simulink model "model"  (R2022b)
settings: Solver=VariableStepAuto  StartTime=0.0  StopTime=15  RelTol=1e-3
libraries: neural x114, simulink x4
(part 3 of 4)

== system model/level=2，训练时间15s，隐藏层30/Layer 2/LW{2,1} ==
  "ad{2,1}" : Inport  PortDimensions=30
      mask Display: e = 0.06;c1 = [120 230 180]/255;c2 = ([120 230 180]+0)/(256+128);c3 = ([120 230 180]+128)/(256+128);patch([0 1 1 0],[0 0 1 1],c1);patch([0 1 1 1-e 1-e 0+e],[0 0 1 1-e 0+e 0+e],c2);patch([0 0 1 1-e 0+e 0+e],[0 1 1 1-e 1-e 0+e],c3);plot([0 1 1 0 0],[0 0 1 1 0]);
  "IW{2,1}(1,:)'" : Constant  Value=[-0.00017015661933175867700888950206916661045397631824016571044921875;-4.93025601643951106906223202930306115376879461109638214111328125e-05;-0.0007115142662295552249129837463215153547935187816619873046875;0.450465904697785302079893199334037490189075469970703125;-0.00035970417057819303353893847230438041151501238346099853515625;-0.00046544183662747154288374940023231829400174319744110107421875;-0.000876727493122407487875780152108973197755403816699981689453125;0.0002626128599686000327818879984675959349260665476322174072265625;0.3370860472746011193834192454232834279537200927734375;-0.00158890258031656596109104651048937739687971770763397216796875;-0.860928350444378320815985716762952506542205810546875;-2.2868367123550593163379407446456070829299278557300567626953125e-05;3.394770767892958175139528353980722386040724813938140869140625e-05;3.60748119126446740024920234457539436334627680480480194091796875e-05;0.00010252607091006281565294389057640955797978676855564117431640625;0.0003053396075934432349514857651939792049233801662921905517578125;-0.0208847293595013257239134674136948888190090656280517578125;0.00018090783389240641491901850912427107687108218669891357421875;0.0035955382769562497201343287400732151581905782222747802734375;2.9147343262242141341718248970238391848397441208362579345703125e-05;-1.044255751802114051685066442587412893772125244140625;7.6663907290150487723601191447642122511751949787139892578125e-05;1.1612112621581929250424991550971753895282745361328125;8.69004399139240257636529474183362253825180232524871826171875e-05;-0.00089584410815050333383446901081015312229283154010772705078125;0.000972428946461849873228455720663987449370324611663818359375;-0.55852210608613506170883056256570853292942047119140625;0.00014495112667725106102116494621867559544625692069530487060546875;-0.0011652466891173842399032078986920168972574174404144287109375;-0.00063093431305860973000443348013277500285767018795013427734375]
      mask Display: e = 0.06;c1 = [120 150 230]/255;c2 = ([120 150 230]+0)/383;c3 = ([120 150 230]+128)/383;patch([0 1 1 0],[0 0 1 1],c1);patch([0 1 1 1-e 1-e 0+e],[0 0 1 1-e 0+e 0+e],c2);patch([0 0 1 1-e 0+e 0+e],[0 1 1 1-e 1-e 0+e],c3);plot([0 1 1 0 0],[0 0 1 1 0]);disp('weights');
  "IW{2,1}(2,:)'" : Constant  Value=[5.38258205100171352648109890370875518783577717840671539306640625e-05;-0.00013672751288354225720177159697499291723943315446376800537109375;0.000678841755202407026725808236733428202569484710693359375;-0.98479814361060780125711744403815828263759613037109375;0.0002569134171630268310103362150442762867896817624568939208984375;0.000626265400513533886280026496962136661750264465808868408203125;0.00056349774478808563153708899307048341142944991588592529296875;-0.000564491732790600199420882887579864473082125186920166015625;-1.2396930325476953616004038849496282637119293212890625;0.00152451867466346234654406277542193492990918457508087158203125;-0.202489611993786733368239083574735559523105621337890625;-0.0004488496149839809744482022058065240344149060547351837158203125;0.0001848497058731152806014541578605303584481589496135711669921875;0.00013099649124499862236185865338455869277822785079479217529296875;-0.000290407580426385570314395945246133123873732984066009521484375;-0.0002539432359679540704248956739519371694768778979778289794921875;0.0241381257840159908767407870300303329713642597198486328125;-0.00025981285471116284668813278813104261644184589385986328125;-0.004254317985620206625518857634915548260323703289031982421875;7.9434875059497178835000996688364693909534253180027008056640625e-05;0.8138138000844878927608760932344011962413787841796875;-0.0002077032004498433558591086178779505644342862069606781005859375;-0.0224187640494880081887263401085874647833406925201416015625;9.7974639247613346903879871785392197125474922358989715576171875e-05;0.00107277211369045423483559176247581490315496921539306640625;-0.00023836869626189699272918176564672876338590867817401885986328125;0.15422244230446391366484704121830873191356658935546875;-0.000510323222761460237699437936242929936270229518413543701171875;0.0013619494124274072154034964654556461027823388576507568359375;0.00018567701461944481947617668904371157623245380818843841552734375]
      mask Display: e = 0.06;c1 = [120 150 230]/255;c2 = ([120 150 230]+0)/383;c3 = ([120 150 230]+128)/383;patch([0 1 1 0],[0 0 1 1],c1);patch([0 1 1 1-e 1-e 0+e],[0 0 1 1-e 0+e 0+e],c2);patch([0 0 1 1-e 0+e 0+e],[0 1 1 1-e 1-e 0+e],c3);plot([0 1 1 0 0],[0 0 1 1 0]);disp('weights');
  Mux : Mux  Inputs=2
      mask Display: e = 0.06;c1 = [120 150 230]/255;c2 = ([120 150 230]+0)/383;c3 = ([120 150 230]+128)/383;patch([0 1 1 0],[0 0 1 1],c1);patch([0 1 1 1-e 1-e 0+e],[0 0 1 1-e 0+e 0+e],c2);patch([0 0 1 1-e 0+e 0+e],[0 1 1 1-e 1-e 0+e],c3);plot([0 1 1 0 0],[0 0 1 1 0]);disp('Mux');
  dotprod1 : neural/Weight Functions/dotprod
  dotprod2 : neural/Weight Functions/dotprod
  "lz{2,1}" : Outport
      mask Display: e = 0.06;c1 = [120 230 180]/255;c2 = ([120 230 180]+0)/(256+128);c3 = ([120 230 180]+128)/(256+128);patch([0 1 1 0],[0 0 1 1],c1);patch([0 1 1 1-e 1-e 0+e],[0 0 1 1-e 0+e 0+e],c2);patch([0 0 1 1-e 0+e 0+e],[0 1 1 1-e 1-e 0+e],c3);plot([0 1 1 0 0],[0 0 1 1 0]);
  wires:
  "IW{2,1}(1,:)'"/1 -> dotprod1/1
  "ad{2,1}"/1 -> dotprod1/2, dotprod2/2
  dotprod1/1 -> Mux/1
  "IW{2,1}(2,:)'"/1 -> dotprod2/1
  dotprod2/1 -> Mux/2
  Mux/1 -> "lz{2,1}"/1

== system model/level=3，训练时间15s，隐藏层15/Layer 1/Delays 1 ==
  "p{1}" : Inport  PortDimensions=12
      mask Display: e = 0.06;c1 = [120 230 180]/255;c2 = ([120 230 180]+0)/(256+128);c3 = ([120 230 180]+128)/(256+128);patch([0 1 1 0],[0 0 1 1],c1);patch([0 1 1 1-e 1-e 0+e],[0 0 1 1-e 0+e 0+e],c2);patch([0 0 1 1-e 0+e 0+e],[0 1 1 1-e 1-e 0+e],c3);plot([0 1 1 0 0],[0 0 1 1 0]);
  mux : Mux  Inputs=1
      mask Display: e = 0.06;c1 = [120 150 230]/255;c2 = ([120 150 230]+0)/383;c3 = ([120 150 230]+128)/383;patch([0 1 1 0],[0 0 1 1],c1);patch([0 1 1 1-e 1-e 0+e],[0 0 1 1-e 0+e 0+e],c2);patch([0 0 1 1-e 0+e 0+e],[0 1 1 1-e 1-e 0+e],c3);plot([0 1 1 0 0],[0 0 1 1 0]);disp('Mux')
  "pd{1,1}" : Outport
      mask Display: e = 0.06;c1 = [120 230 180]/255;c2 = ([120 230 180]+0)/(256+128);c3 = ([120 230 180]+128)/(256+128);patch([0 1 1 0],[0 0 1 1],c1);patch([0 1 1 1-e 1-e 0+e],[0 0 1 1-e 0+e 0+e],c2);patch([0 0 1 1-e 0+e 0+e],[0 1 1 1-e 1-e 0+e],c3);plot([0 1 1 0 0],[0 0 1 1 0]);
  wires:
  "p{1}"/1 -> mux/1
  mux/1 -> "pd{1,1}"/1

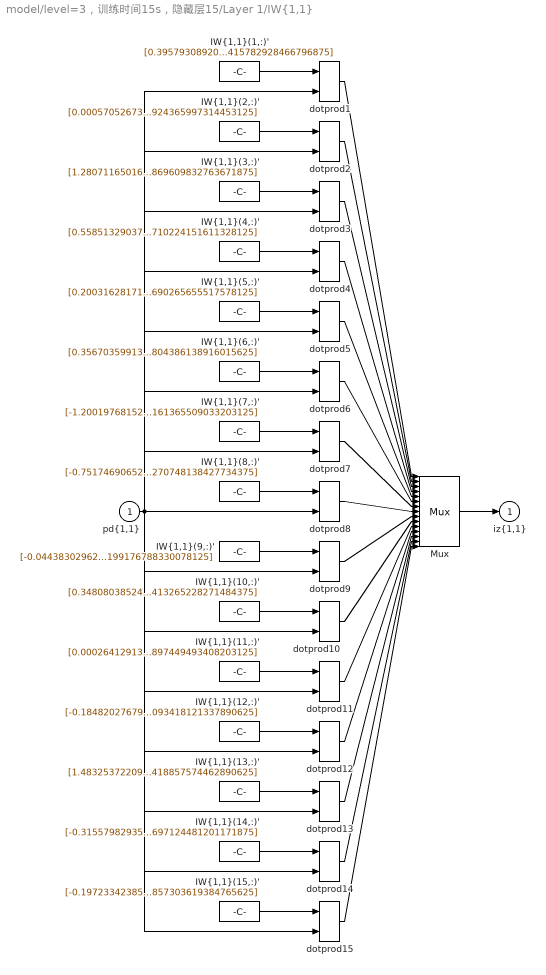
== system model/level=3，训练时间15s，隐藏层15/Layer 1/IW{1,1} ==
  "pd{1,1}" : Inport  PortDimensions=12
      mask Display: e = 0.06;c1 = [120 230 180]/255;c2 = ([120 230 180]+0)/(256+128);c3 = ([120 230 180]+128)/(256+128);patch([0 1 1 0],[0 0 1 1],c1);patch([0 1 1 1-e 1-e 0+e],[0 0 1 1-e 0+e 0+e],c2);patch([0 0 1 1-e 0+e 0+e],[0 1 1 1-e 1-e 0+e],c3);plot([0 1 1 0 0],[0 0 1 1 0]);
  "IW{1,1}(1,:)'" : Constant  Value=[0.3957930892014740464901478844694793224334716796875;0.086698682741434496268340126334805972874164581298828125;0.057978420610327340012357666410025558434426784515380859375;-0.11708503503631663422712705369121977128088474273681640625;0.5757139566791853457772276669857092201709747314453125;0.100001463605383589250408249426982365548610687255859375;-0.360494014120566863557115766525384970009326934814453125;0.331018839262216479912837030497030355036258697509765625;0.67861213442945389484606266705668531358242034912109375;1.62287556740570426683234472875483334064483642578125;1.1914706007323612180215377520653419196605682373046875;1.5007337994294249750026892797905020415782928466796875]
      mask Display: e = 0.06;c1 = [120 150 230]/255;c2 = ([120 150 230]+0)/383;c3 = ([120 150 230]+128)/383;patch([0 1 1 0],[0 0 1 1],c1);patch([0 1 1 1-e 1-e 0+e],[0 0 1 1-e 0+e 0+e],c2);patch([0 0 1 1-e 0+e 0+e],[0 1 1 1-e 1-e 0+e],c3);plot([0 1 1 0 0],[0 0 1 1 0]);disp('Weights');
  "IW{1,1}(10,:)'" : Constant  Value=[0.348080385247078794019870429110596887767314910888671875;-2.255687632373656992257338060881011188030242919921875;-0.8917795900077691850782457549939863383769989013671875;1.1584959880156178169130498645245097577571868896484375;-0.81101211177083321057779130569542758166790008544921875;0.062260937313953899907570388450039899908006191253662109375;0.53574182001364734073689533033757470548152923583984375;-0.2128709739492778696412500494261621497571468353271484375;-0.46279511588180832770689221433713100850582122802734375;-0.34533064631210741435296540657873265445232391357421875;-1.10111951608478175756999917211942374706268310546875;1.12329307949009571387932737707160413265228271484375]
      mask Display: e = 0.06;c1 = [120 150 230]/255;c2 = ([120 150 230]+0)/383;c3 = ([120 150 230]+128)/383;patch([0 1 1 0],[0 0 1 1],c1);patch([0 1 1 1-e 1-e 0+e],[0 0 1 1-e 0+e 0+e],c2);patch([0 0 1 1-e 0+e 0+e],[0 1 1 1-e 1-e 0+e],c3);plot([0 1 1 0 0],[0 0 1 1 0]);disp('Weights');
  "IW{1,1}(11,:)'" : Constant  Value=[0.0002641291373141290798991220878377816916326992213726043701171875;1.69280234455796972669640310105165781351388432085514068603515625e-05;0.00059389072570711367270168690168929970241151750087738037109375;0.000817075702284870562970564566995790301007218658924102783203125;-0.0002773395932363266892621556092279888616758398711681365966796875;0.000419950685599850752176276369453944425913505256175994873046875;1.7279375298931984872297107358463108539581298828125;1.1830523399036094733816071311593987047672271728515625;0.385067347353057087833150262667913921177387237548828125;0.47274192642379031514821008386206813156604766845703125;-0.85106281929793781149129472396452911198139190673828125;-0.75527215984610063248538835978251881897449493408203125]
      mask Display: e = 0.06;c1 = [120 150 230]/255;c2 = ([120 150 230]+0)/383;c3 = ([120 150 230]+128)/383;patch([0 1 1 0],[0 0 1 1],c1);patch([0 1 1 1-e 1-e 0+e],[0 0 1 1-e 0+e 0+e],c2);patch([0 0 1 1-e 0+e 0+e],[0 1 1 1-e 1-e 0+e],c3);plot([0 1 1 0 0],[0 0 1 1 0]);disp('Weights');
  "IW{1,1}(12,:)'" : Constant  Value=[-0.1848202767977935312426751579550909809768199920654296875;0.012338003346249258596056819214936695061624050140380859375;0.09999923402391842908176755599924945272505283355712890625;-0.29923701483788744948100202236673794686794281005859375;-0.2017986819280386534547488963653449900448322296142578125;-0.00197252352955649447319164124792223447002470493316650390625;-1.370526397980648791730118318810127675533294677734375;-0.58819022085026995139145356006338261067867279052734375;-0.8059703463854150928824537913897074759006500244140625;0.602810685508602173143799518584273755550384521484375;0.87530414850278026595020719469175674021244049072265625;-0.00901182558217848185544429640003727399744093418121337890625]
      mask Display: e = 0.06;c1 = [120 150 230]/255;c2 = ([120 150 230]+0)/383;c3 = ([120 150 230]+128)/383;patch([0 1 1 0],[0 0 1 1],c1);patch([0 1 1 1-e 1-e 0+e],[0 0 1 1-e 0+e 0+e],c2);patch([0 0 1 1-e 0+e 0+e],[0 1 1 1-e 1-e 0+e],c3);plot([0 1 1 0 0],[0 0 1 1 0]);disp('Weights');
  "IW{1,1}(13,:)'" : Constant  Value=[1.4832537220993196047658102543209679424762725830078125;0.206296960918707750209932783036492764949798583984375;-0.86180429757193277584548241065931506454944610595703125;-0.52558132261974599419573905834113247692584991455078125;1.22454643654238193306582616060040891170501708984375;0.64085174940409228572235633691889233887195587158203125;1.730080809760341953307261064765043556690216064453125;4.73501628594810686223581797094084322452545166015625;2.770509814033699225177542757592163980007171630859375;2.547005844747089131629991243244148790836334228515625;2.063288887946004734885718789882957935333251953125;0.56434669201611209476965314024710096418857574462890625]
      mask Display: e = 0.06;c1 = [120 150 230]/255;c2 = ([120 150 230]+0)/383;c3 = ([120 150 230]+128)/383;patch([0 1 1 0],[0 0 1 1],c1);patch([0 1 1 1-e 1-e 0+e],[0 0 1 1-e 0+e 0+e],c2);patch([0 0 1 1-e 0+e 0+e],[0 1 1 1-e 1-e 0+e],c3);plot([0 1 1 0 0],[0 0 1 1 0]);disp('Weights');
  "IW{1,1}(14,:)'" : Constant  Value=[-0.315579829351021301508950500647188164293766021728515625;-0.446476214520890035686306873685680329799652099609375;0.11181665067909492272679727875583921559154987335205078125;-0.1734197577485878383196649110686848871409893035888671875;-0.55458424585295273967489038113853894174098968505859375;-0.00713583417339959912017999243971644318662583827972412109375;0.523121900009196227898655706667341291904449462890625;-0.90958149150058964504950154150719754397869110107421875;-0.477576994671569388106746600897167809307575225830078125;-0.83211716086969167438525118996039964258670806884765625;-2.466955793154146814316618474549613893032073974609375;-0.319842229521164866934412884802441112697124481201171875]
      mask Display: e = 0.06;c1 = [120 150 230]/255;c2 = ([120 150 230]+0)/383;c3 = ([120 150 230]+128)/383;patch([0 1 1 0],[0 0 1 1],c1);patch([0 1 1 1-e 1-e 0+e],[0 0 1 1-e 0+e 0+e],c2);patch([0 0 1 1-e 0+e 0+e],[0 1 1 1-e 1-e 0+e],c3);plot([0 1 1 0 0],[0 0 1 1 0]);disp('Weights');
  "IW{1,1}(15,:)'" : Constant  Value=[-0.197233423851313094399273495582747273147106170654296875;0.5473786302866192610139250973588787019252777099609375;-0.725643644094891016038673114962875843048095703125;-0.88789741317147352628325052137370221316814422607421875;1.2322632390997310114499896371853537857532501220703125;-0.115690710417836573054017890171962790191173553466796875;-0.1614833249582365570784503461254644207656383514404296875;-2.646540132170490000618201520410366356372833251953125;-1.9052574260331194277995336960884742438793182373046875;0.433805464346474212167237283210852183401584625244140625;0.1976267970320291500474496615424868650734424591064453125;0.96546430930502058487263639108277857303619384765625]
      mask Display: e = 0.06;c1 = [120 150 230]/255;c2 = ([120 150 230]+0)/383;c3 = ([120 150 230]+128)/383;patch([0 1 1 0],[0 0 1 1],c1);patch([0 1 1 1-e 1-e 0+e],[0 0 1 1-e 0+e 0+e],c2);patch([0 0 1 1-e 0+e 0+e],[0 1 1 1-e 1-e 0+e],c3);plot([0 1 1 0 0],[0 0 1 1 0]);disp('Weights');
  "IW{1,1}(2,:)'" : Constant  Value=[0.00057052673433711478985508325223463543807156383991241455078125;0.000104860431229279643162467794414993704776861704885959625244140625;-0.00133157910874800631227665714817476327880285680294036865234375;0.00118649266440457143607922763095530171995051205158233642578125;0.000118536181079970996091361989943635535382782109081745147705078125;0.000560127271953092423055486914762468586559407413005828857421875;-2.02499596832077077834810552303679287433624267578125;-1.5218905321397315777431913375039584934711456298828125;-1.471139301702704127450260784826241433620452880859375;-0.7543825893970026452706179043161682784557342529296875;1.6585879615043468415791494408040307462215423583984375;0.96620580919715781664791620642063207924365997314453125]
      mask Display: e = 0.06;c1 = [120 150 230]/255;c2 = ([120 150 230]+0)/383;c3 = ([120 150 230]+128)/383;patch([0 1 1 0],[0 0 1 1],c1);patch([0 1 1 1-e 1-e 0+e],[0 0 1 1-e 0+e 0+e],c2);patch([0 0 1 1-e 0+e 0+e],[0 1 1 1-e 1-e 0+e],c3);plot([0 1 1 0 0],[0 0 1 1 0]);disp('Weights');
  "IW{1,1}(3,:)'" : Constant  Value=[1.280711650164423787146006361581385135650634765625;-0.418703333982376191269025866859010420739650726318359375;0.01268262333086577452190280013155643246136605739593505859375;1.406475454930298241151831462047994136810302734375;-0.39942954805115393757120045847841538488864898681640625;-0.53036973140369070289779074300895445048809051513671875;-3.426049819494218606763524803682230412960052490234375;2.38266649232553806569967491668649017810821533203125;0.66860167569183304170366000107605941593647003173828125;-0.81667720428670509402735433468478731811046600341796875;1.85509852622451898440658624167554080486297607421875;-3.262343835552200754790419523487798869609832763671875]
      mask Display: e = 0.06;c1 = [120 150 230]/255;c2 = ([120 150 230]+0)/383;c3 = ([120 150 230]+128)/383;patch([0 1 1 0],[0 0 1 1],c1);patch([0 1 1 1-e 1-e 0+e],[0 0 1 1-e 0+e 0+e],c2);patch([0 0 1 1-e 0+e 0+e],[0 1 1 1-e 1-e 0+e],c3);plot([0 1 1 0 0],[0 0 1 1 0]);disp('Weights');
  "IW{1,1}(4,:)'" : Constant  Value=[0.55851329037293029333710592254647053778171539306640625;0.314383357949808928122337192689883522689342498779296875;-0.2916339194998922579316058545373380184173583984375;0.480482703452632720075854422248085029423236846923828125;-0.324142221104775030138256397549412213265895843505859375;0.623133017290093516038496090914122760295867919921875;0.60798485222378062520220964870532043278217315673828125;-0.89992032388483778060361828465829603374004364013671875;-0.2443731124429557866051254677586257457733154296875;0.280039630981737008852405779180116951465606689453125;0.79383226740657375497534076203010044991970062255859375;0.362518261297716748448038970309426076710224151611328125]
      mask Display: e = 0.06;c1 = [120 150 230]/255;c2 = ([120 150 230]+0)/383;c3 = ([120 150 230]+128)/383;patch([0 1 1 0],[0 0 1 1],c1);patch([0 1 1 1-e 1-e 0+e],[0 0 1 1-e 0+e 0+e],c2);patch([0 0 1 1-e 0+e 0+e],[0 1 1 1-e 1-e 0+e],c3);plot([0 1 1 0 0],[0 0 1 1 0]);disp('Weights');
  "IW{1,1}(5,:)'" : Constant  Value=[0.2003162817142581098028841779523645527660846710205078125;-0.300298530088698167883620726570370607078075408935546875;-0.61941573448953379799064578037359751760959625244140625;0.2341949148435984728866543491676566191017627716064453125;0.11315803139559747758635666059490176849067211151123046875;0.2405047482176067286108178677750402130186557769775390625;0.0427712090246665510573365054369787685573101043701171875;-1.2505725621219634380310026244842447340488433837890625;-0.52172280362525025321218663520994596183300018310546875;0.3388856987794832686944346278323791921138763427734375;-1.0048096488192308495257520917220972478389739990234375;0.301074262734163433652412322771851904690265655517578125]
      mask Display: e = 0.06;c1 = [120 150 230]/255;c2 = ([120 150 230]+0)/383;c3 = ([120 150 230]+128)/383;patch([0 1 1 0],[0 0 1 1],c1);patch([0 1 1 1-e 1-e 0+e],[0 0 1 1-e 0+e 0+e],c2);patch([0 0 1 1-e 0+e 0+e],[0 1 1 1-e 1-e 0+e],c3);plot([0 1 1 0 0],[0 0 1 1 0]);disp('Weights');
  "IW{1,1}(6,:)'" : Constant  Value=[0.356703599139141402929453761316835880279541015625;0.03235781593064350480926094633105094544589519500732421875;-0.35394747297565587462742087154765613377094268798828125;0.31792719784468836952129322526161558926105499267578125;0.4828265406684224547717576569993980228900909423828125;-0.483511938086240267153925742604769766330718994140625;-0.6867746666480123440834404391353018581867218017578125;-0.81450304831739106514731929564732126891613006591796875;-0.7627521791053315514119503859546966850757598876953125;-0.80021919178302081121501032612286508083343505859375;0.1280786866916479305178455661007319577038288116455078125;-0.792028304453565201725950828404165804386138916015625]
      mask Display: e = 0.06;c1 = [120 150 230]/255;c2 = ([120 150 230]+0)/383;c3 = ([120 150 230]+128)/383;patch([0 1 1 0],[0 0 1 1],c1);patch([0 1 1 1-e 1-e 0+e],[0 0 1 1-e 0+e 0+e],c2);patch([0 0 1 1-e 0+e 0+e],[0 1 1 1-e 1-e 0+e],c3);plot([0 1 1 0 0],[0 0 1 1 0]);disp('Weights');
  "IW{1,1}(7,:)'" : Constant  Value=[-1.2001976815232295287103232717118572736580972559750080108642578125e-05;0.000118348687342715078694987962393270208849571645259857177734375;-0.00024302797422544485301566796753292010180302895605564117431640625;-0.0004555539671597588356928565378467510527116246521472930908203125;0.000134278757741061456447428934524168653297238051891326904296875;-0.00021405521769952661468618126949792213054024614393711090087890625;-0.65831716300174292211266902086208574473857879638671875;-0.92289898350056376319372475336422212421894073486328125;-0.452783051231515243362224509837687946856021881103515625;-0.1198156760386257235762030859405058436095714569091796875;0.5356858778913728968973373412154614925384521484375;0.398703493317783153049305155946058221161365509033203125]
      mask Display: e = 0.06;c1 = [120 150 230]/255;c2 = ([120 150 230]+0)/383;c3 = ([120 150 230]+128)/383;patch([0 1 1 0],[0 0 1 1],c1);patch([0 1 1 1-e 1-e 0+e],[0 0 1 1-e 0+e 0+e],c2);patch([0 0 1 1-e 0+e 0+e],[0 1 1 1-e 1-e 0+e],c3);plot([0 1 1 0 0],[0 0 1 1 0]);disp('Weights');
  "IW{1,1}(8,:)'" : Constant  Value=[-0.75174690652320996786528439770336262881755828857421875;-0.0904724174773055833664869851418188773095607757568359375;-0.212599975995264423023201061369036324322223663330078125;0.320182849608710962119317855467670597136020660400390625;0.06106449733927120371301811019293381832540035247802734375;-0.841963820469229684562151305726729333400726318359375;1.1622486606228712435751049270038492977619171142578125;-1.3389692521529090729615063537494279444217681884765625;-0.72122321356091279032085594735690392553806304931640625;-0.54314731395936444169336709819617681205272674560546875;-0.2696144951149055390970943335560150444507598876953125;-0.500567157778385674049559384002350270748138427734375]
      mask Display: e = 0.06;c1 = [120 150 230]/255;c2 = ([120 150 230]+0)/383;c3 = ([120 150 230]+128)/383;patch([0 1 1 0],[0 0 1 1],c1);patch([0 1 1 1-e 1-e 0+e],[0 0 1 1-e 0+e 0+e],c2);patch([0 0 1 1-e 0+e 0+e],[0 1 1 1-e 1-e 0+e],c3);plot([0 1 1 0 0],[0 0 1 1 0]);disp('Weights');
  "IW{1,1}(9,:)'" : Constant  Value=[-0.0443830296271111313100021789068705402314662933349609375;0.01477298965334654379244483379807206802070140838623046875;0.0182822479157221419454604216525694937445223331451416015625;0.020633462184774860326275103261650656349956989288330078125;-0.249316620626878648891988632385618984699249267578125;0.05863171649468214285949585473645129241049289703369140625;-1.7838935545885903355411983284284360706806182861328125;-3.060798654660634721125234136707149446010589599609375;-1.3841554952636554443046179585508070886135101318359375;-0.69048528742817882886129154940135776996612548828125;-0.463179700521488879605414012985420413315296173095703125;-0.0977294875845675925507549663961981423199176788330078125]
      mask Display: e = 0.06;c1 = [120 150 230]/255;c2 = ([120 150 230]+0)/383;c3 = ([120 150 230]+128)/383;patch([0 1 1 0],[0 0 1 1],c1);patch([0 1 1 1-e 1-e 0+e],[0 0 1 1-e 0+e 0+e],c2);patch([0 0 1 1-e 0+e 0+e],[0 1 1 1-e 1-e 0+e],c3);plot([0 1 1 0 0],[0 0 1 1 0]);disp('Weights');
  Mux : Mux  Inputs=15
      mask Display: e = 0.06;c1 = [120 150 230]/255;c2 = ([120 150 230]+0)/383;c3 = ([120 150 230]+128)/383;patch([0 1 1 0],[0 0 1 1],c1);patch([0 1 1 1-e 1-e 0+e],[0 0 1 1-e 0+e 0+e],c2);patch([0 0 1 1-e 0+e 0+e],[0 1 1 1-e 1-e 0+e],c3);plot([0 1 1 0 0],[0 0 1 1 0]);disp('Mux');
  dotprod{1..15} (15 alike) : neural/Weight Functions/dotprod
  "iz{1,1}" : Outport
      mask Display: e = 0.06;c1 = [120 230 180]/255;c2 = ([120 230 180]+0)/(256+128);c3 = ([120 230 180]+128)/(256+128);patch([0 1 1 0],[0 0 1 1],c1);patch([0 1 1 1-e 1-e 0+e],[0 0 1 1-e 0+e 0+e],c2);patch([0 0 1 1-e 0+e 0+e],[0 1 1 1-e 1-e 0+e],c3);plot([0 1 1 0 0],[0 0 1 1 0]);
  wires:
  "IW{1,1}(1,:)'"/1 -> dotprod1/1
  "pd{1,1}"/1 -> dotprod1/2, dotprod2/2, dotprod3/2, dotprod4/2, dotprod5/2, dotprod6/2, dotprod7/2, dotprod8/2, dotprod9/2, dotprod10/2, dotprod11/2, dotprod12/2, dotprod13/2, dotprod14/2, dotprod15/2
  dotprod1/1 -> Mux/1
  "IW{1,1}(2,:)'"/1 -> dotprod2/1
  dotprod2/1 -> Mux/2
  "IW{1,1}(3,:)'"/1 -> dotprod3/1
  dotprod3/1 -> Mux/3
  "IW{1,1}(4,:)'"/1 -> dotprod4/1
  dotprod4/1 -> Mux/4
  "IW{1,1}(5,:)'"/1 -> dotprod5/1
  dotprod5/1 -> Mux/5
  "IW{1,1}(6,:)'"/1 -> dotprod6/1
  dotprod6/1 -> Mux/6
  "IW{1,1}(7,:)'"/1 -> dotprod7/1
  dotprod7/1 -> Mux/7
  "IW{1,1}(8,:)'"/1 -> dotprod8/1
  dotprod8/1 -> Mux/8
  "IW{1,1}(9,:)'"/1 -> dotprod9/1
  dotprod9/1 -> Mux/9
  "IW{1,1}(10,:)'"/1 -> dotprod10/1
  dotprod10/1 -> Mux/10
  "IW{1,1}(11,:)'"/1 -> dotprod11/1
  dotprod11/1 -> Mux/11
  "IW{1,1}(12,:)'"/1 -> dotprod12/1
  dotprod12/1 -> Mux/12
  "IW{1,1}(13,:)'"/1 -> dotprod13/1
  dotprod13/1 -> Mux/13
  "IW{1,1}(14,:)'"/1 -> dotprod14/1
  dotprod14/1 -> Mux/14
  "IW{1,1}(15,:)'"/1 -> dotprod15/1
  dotprod15/1 -> Mux/15
  Mux/1 -> "iz{1,1}"/1

== system model/level=3，训练时间15s，隐藏层15/Layer 2/Delays 1 ==
  "p{2}" : Inport  PortDimensions=15
      mask Display: e = 0.06;c1 = [120 230 180]/255;c2 = ([120 230 180]+0)/(256+128);c3 = ([120 230 180]+128)/(256+128);patch([0 1 1 0],[0 0 1 1],c1);patch([0 1 1 1-e 1-e 0+e],[0 0 1 1-e 0+e 0+e],c2);patch([0 0 1 1-e 0+e 0+e],[0 1 1 1-e 1-e 0+e],c3);plot([0 1 1 0 0],[0 0 1 1 0]);
  mux : Mux  Inputs=1
      mask Display: e = 0.06;c1 = [120 150 230]/255;c2 = ([120 150 230]+0)/383;c3 = ([120 150 230]+128)/383;patch([0 1 1 0],[0 0 1 1],c1);patch([0 1 1 1-e 1-e 0+e],[0 0 1 1-e 0+e 0+e],c2);patch([0 0 1 1-e 0+e 0+e],[0 1 1 1-e 1-e 0+e],c3);plot([0 1 1 0 0],[0 0 1 1 0]);disp('Mux')
  "pd{2,1}" : Outport
      mask Display: e = 0.06;c1 = [120 230 180]/255;c2 = ([120 230 180]+0)/(256+128);c3 = ([120 230 180]+128)/(256+128);patch([0 1 1 0],[0 0 1 1],c1);patch([0 1 1 1-e 1-e 0+e],[0 0 1 1-e 0+e 0+e],c2);patch([0 0 1 1-e 0+e 0+e],[0 1 1 1-e 1-e 0+e],c3);plot([0 1 1 0 0],[0 0 1 1 0]);
  wires:
  "p{2}"/1 -> mux/1
  mux/1 -> "pd{2,1}"/1

== system model/level=3，训练时间15s，隐藏层15/Layer 2/LW{2,1} ==
  "ad{2,1}" : Inport  PortDimensions=15
      mask Display: e = 0.06;c1 = [120 230 180]/255;c2 = ([120 230 180]+0)/(256+128);c3 = ([120 230 180]+128)/(256+128);patch([0 1 1 0],[0 0 1 1],c1);patch([0 1 1 1-e 1-e 0+e],[0 0 1 1-e 0+e 0+e],c2);patch([0 0 1 1-e 0+e 0+e],[0 1 1 1-e 1-e 0+e],c3);plot([0 1 1 0 0],[0 0 1 1 0]);
  "IW{2,1}(1,:)'" : Constant  Value=[-0.000583166795668617018479074065595568754361011087894439697265625;-0.94518166305313588981817929379758425056934356689453125;-0.0001660050785545720748205555938881161637254990637302398681640625;-0.0001070859157649753888585930639010257436893880367279052734375;0.0003842390015297906494425028700590019070659764111042022705078125;-0.00141413989882815623912171165699191988096572458744049072265625;3.06609074067634512772428934113122522830963134765625;0.000321304946913954160743476240469362892326898872852325439453125;-0.002507133529169654206913975258430582471191883087158203125;-5.79899779198733041616665995210411210791789926588535308837890625e-05;1.95202779060717812598113596322946250438690185546875;-0.00427473866415701946042116077251193928532302379608154296875;0.00014032622636912125383031046954585008279536850750446319580078125;0.000529871576981954194550394898755030226311646401882171630859375;0.000281771872796035094226041461951126620988361537456512451171875]
      mask Display: e = 0.06;c1 = [120 150 230]/255;c2 = ([120 150 230]+0)/383;c3 = ([120 150 230]+128)/383;patch([0 1 1 0],[0 0 1 1],c1);patch([0 1 1 1-e 1-e 0+e],[0 0 1 1-e 0+e 0+e],c2);patch([0 0 1 1-e 0+e 0+e],[0 1 1 1-e 1-e 0+e],c3);plot([0 1 1 0 0],[0 0 1 1 0]);disp('weights');
  "IW{2,1}(2,:)'" : Constant  Value=[0.000629268742799666928877666549624336767010390758514404296875;0.8431479968246005096688122648629359900951385498046875;5.283054698854418806085175841502632465562783181667327880859375e-05;-9.28822901168978678522469838441111278370954096317291259765625e-05;-0.000500904251595419669311481936091468014637939631938934326171875;0.0015103274817080953977554980127706585335545241832733154296875;-4.28475774020505273398384815664030611515045166015625;-0.00018959665540160534793860669378062766554648987948894500732421875;0.0003261444294967476829373576041604110287153162062168121337890625;6.2049605053103649814072451107449523988179862499237060546875e-05;-1.743219041318246009808490271097980439662933349609375;0.004226542359433101136989563428869587369263172149658203125;-5.891125076672439433468630998191883918480016291141510009765625e-05;-0.000804979871354513112045869771549178040004335343837738037109375;0.0001707441112262775002698933501932287981617264449596405029296875]
      mask Display: e = 0.06;c1 = [120 150 230]/255;c2 = ([120 150 230]+0)/383;c3 = ([120 150 230]+128)/383;patch([0 1 1 0],[0 0 1 1],c1);patch([0 1 1 1-e 1-e 0+e],[0 0 1 1-e 0+e 0+e],c2);patch([0 0 1 1-e 0+e 0+e],[0 1 1 1-e 1-e 0+e],c3);plot([0 1 1 0 0],[0 0 1 1 0]);disp('weights');
  Mux : Mux  Inputs=2
      mask Display: e = 0.06;c1 = [120 150 230]/255;c2 = ([120 150 230]+0)/383;c3 = ([120 150 230]+128)/383;patch([0 1 1 0],[0 0 1 1],c1);patch([0 1 1 1-e 1-e 0+e],[0 0 1 1-e 0+e 0+e],c2);patch([0 0 1 1-e 0+e 0+e],[0 1 1 1-e 1-e 0+e],c3);plot([0 1 1 0 0],[0 0 1 1 0]);disp('Mux');
  dotprod1 : neural/Weight Functions/dotprod
  dotprod2 : neural/Weight Functions/dotprod
  "lz{2,1}" : Outport
      mask Display: e = 0.06;c1 = [120 230 180]/255;c2 = ([120 230 180]+0)/(256+128);c3 = ([120 230 180]+128)/(256+128);patch([0 1 1 0],[0 0 1 1],c1);patch([0 1 1 1-e 1-e 0+e],[0 0 1 1-e 0+e 0+e],c2);patch([0 0 1 1-e 0+e 0+e],[0 1 1 1-e 1-e 0+e],c3);plot([0 1 1 0 0],[0 0 1 1 0]);
  wires:
  "IW{2,1}(1,:)'"/1 -> dotprod1/1
  "ad{2,1}"/1 -> dotprod1/2, dotprod2/2
  dotprod1/1 -> Mux/1
  "IW{2,1}(2,:)'"/1 -> dotprod2/1
  dotprod2/1 -> Mux/2
  Mux/1 -> "lz{2,1}"/1

== system model/level=3，训练时间15s，隐藏层30/Layer 1/Delays 1 ==
  "p{1}" : Inport  PortDimensions=12
      mask Display: e = 0.06;c1 = [120 230 180]/255;c2 = ([120 230 180]+0)/(256+128);c3 = ([120 230 180]+128)/(256+128);patch([0 1 1 0],[0 0 1 1],c1);patch([0 1 1 1-e 1-e 0+e],[0 0 1 1-e 0+e 0+e],c2);patch([0 0 1 1-e 0+e 0+e],[0 1 1 1-e 1-e 0+e],c3);plot([0 1 1 0 0],[0 0 1 1 0]);
  mux : Mux  Inputs=1
      mask Display: e = 0.06;c1 = [120 150 230]/255;c2 = ([120 150 230]+0)/383;c3 = ([120 150 230]+128)/383;patch([0 1 1 0],[0 0 1 1],c1);patch([0 1 1 1-e 1-e 0+e],[0 0 1 1-e 0+e 0+e],c2);patch([0 0 1 1-e 0+e 0+e],[0 1 1 1-e 1-e 0+e],c3);plot([0 1 1 0 0],[0 0 1 1 0]);disp('Mux')
  "pd{1,1}" : Outport
      mask Display: e = 0.06;c1 = [120 230 180]/255;c2 = ([120 230 180]+0)/(256+128);c3 = ([120 230 180]+128)/(256+128);patch([0 1 1 0],[0 0 1 1],c1);patch([0 1 1 1-e 1-e 0+e],[0 0 1 1-e 0+e 0+e],c2);patch([0 0 1 1-e 0+e 0+e],[0 1 1 1-e 1-e 0+e],c3);plot([0 1 1 0 0],[0 0 1 1 0]);
  wires:
  "p{1}"/1 -> mux/1
  mux/1 -> "pd{1,1}"/1
